simulink model "simulink_ej1"  (R2021a)
settings: Solver=FixedStepAuto  StartTime=0.0  StopTime=5.0  FixedStep=0.02  RelTol=1e-3
libraries: roblocks x1
settings Model: Creator=santi  LastModifiedBy=omsma

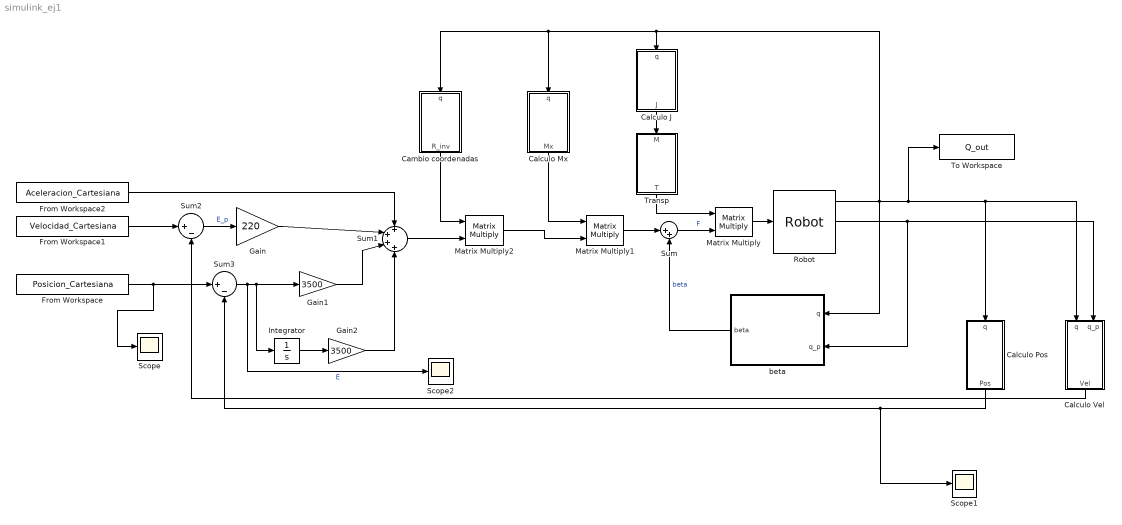
== system simulink_ej1 ==
  Calculo J : MATLAB Function  TreatAsAtomicUnit=on
  Calculo Mx : MATLAB Function  TreatAsAtomicUnit=on
  Calculo Pos : MATLAB Function  TreatAsAtomicUnit=on
  Calculo Vel : MATLAB Function  TreatAsAtomicUnit=on
  Cambio coordenadas : MATLAB Function  TreatAsAtomicUnit=on
  From Workspace : FromWorkspace  VariableName=Posicion_Cartesiana  SampleTime=-1
  From Workspace1 : FromWorkspace  VariableName=Velocidad_Cartesiana  SampleTime=-1
  From Workspace2 : FromWorkspace  VariableName=Aceleracion_Cartesiana  SampleTime=-1
  Gain : Gain  Gain=220
  Gain1 : Gain  Gain=3500
  Gain2 : Gain  Gain=3500
  Integrator : Integrator
  Matrix Multiply : Product  Multiplication=Matrix(*)
  Matrix Multiply1 : Product  Multiplication=Matrix(*)
  Matrix Multiply2 : Product  Multiplication=Matrix(*)
  Robot : roblocks/Arm/Robot  robot=rob  q0=[0, -pi/2]
  Scope : Scope
  Scope1 : Scope
  Scope2 : Scope
  Sum : Sum  Inputs=|++
  Sum1 : Sum  Inputs=++++
  Sum2 : Sum  Inputs=|+-
  Sum3 : Sum  Inputs=|+-
  To Workspace : ToWorkspace  VariableName=Q_out  SampleTime=-1
      settings: Save2DSignal=2-D array (concatenate along first dimension)
  Transp : MATLAB Function  TreatAsAtomicUnit=on
  beta : MATLAB Function  TreatAsAtomicUnit=on
  wires:
  Transp/1(T) -> Matrix Multiply/1
  Calculo Vel/1(Vel) -> Sum2/2
  Calculo Pos/1(Pos) -> Scope1/1, Sum3/2
  Calculo J/1(J) -> Transp/1(M)
  Calculo Mx/1(Mx) -> Matrix Multiply1/1
  Matrix Multiply1/1 -> Sum/1
  Robot/1 -> beta/1(q), Calculo J/1(q), Cambio coordenadas/1(q), Calculo Mx/1(q), Calculo Vel/1(q), Calculo Pos/1(q), To Workspace/1
  Robot/2 -> Calculo Vel/2(q_p), beta/2(q_p)
  beta/1(beta) -> Sum/2  "beta"
  Matrix Multiply2/1 -> Matrix Multiply1/2
  Sum2/1 -> Gain/1  "E_p"
  Sum/1 -> Matrix Multiply/2  "F"
  Cambio coordenadas/1(R_inv) -> Matrix Multiply2/1
  Matrix Multiply/1 -> Robot/1
  Gain1/1 -> Sum1/3
  From Workspace2/1 -> Sum1/1
  From Workspace1/1 -> Sum2/1
  Gain/1 -> Sum1/2
  From Workspace/1 -> Scope/1, Sum3/1
  Sum3/1 -> Scope2/1, Integrator/1, Gain1/1  "E"
  Sum1/1 -> Matrix Multiply2/2
  Integrator/1 -> Gain2/1
  Gain2/1 -> Sum1/4

== matlab function simulink_ej1/Cambio coordenadas ==
  data: q input; R_inv output
function R_inv = R_inv(q)

t1 = q(1);
t2 = q(2);

R_inv = [cos(t1+t2), sin(t1+t2); -sin(t1+t2), cos(t1+t2)];

== matlab function simulink_ej1/Transp ==
  data: M input; T output
function T = T(M)

T = M';

== matlab function simulink_ej1/beta ==
  data: q input; beta output; q_p input
function beta = beta(q, q_p)
%#codegen
coder.extrinsic('gravload_wrapper');
coder.extrinsic('friction_wrapper');
coder.extrinsic('coriolis_wrapper');

% Preasignaciones
beta = zeros(2,1);
rG = zeros(2,1);
rF = zeros(2,1);
rC = zeros(2,2);
rV = zeros(2,1);


% Llamadas extrínsecas (Simulink ejecutará en MATLAB)
rG = gravload_wrapper([q(1), q(2)]);
rF = friction_wrapper([q_p(1), q_p(2)]);
rC = coriolis_wrapper([q(1), q(2)], [q_p(1), q_p(2)]);

% Cálculos locales
rV = rC * q_p;
beta = rG + rV + rF;
end

== matlab function simulink_ej1/Calculo Mx ==
  data: q input; Mx output
function Mx = Mx(q)

t1 = q(1);
t2 = q(2);

Mx = [(2-cos(t2)^2)/(sin(t2)^2), 0; 0,  1];

== matlab function simulink_ej1/Calculo Pos ==
  data: q input; Pos output
function Pos = Pos(q)

t1 = q(1);
t2 = q(2);

Pos = [cos(t1+t2) + cos(t1); sin(t1+t2) + sin(t1)];

== matlab function simulink_ej1/Calculo Vel ==
  data: q input; Vel output; q_p input
function Vel = Vel(q, q_p)

t1 = q(1);
t2 = q(2);

t1_p = q_p(1);
t2_p = q_p(2);

R = [cos(t1+t2), -sin(t1+t2); 
     sin(t1+t2), cos(t1+t2)];
 
v = [sin(t2)*t1_p; cos(t2)*t1_p];
 
wxp = [0; t1_p+t2_p];

Vel = R*(v + wxp);

== matlab function simulink_ej1/Calculo J ==
  data: q input; J output
function J = J(q)

t1 = q(1);
t2 = q(2);

J = [sin(t2) 0; cos(t2)+1 1];
